simulink model "DT_PID"  (R2025b)
settings: Solver=ode4  StartTime=0.0  StopTime=10.0  FixedStep=0.01  RelTol=1e-3
model workspace (MAT data in the model file):
  K = 126
  tau = 0.1
settings Model: Creator=joshc  LastModifiedBy=joshc

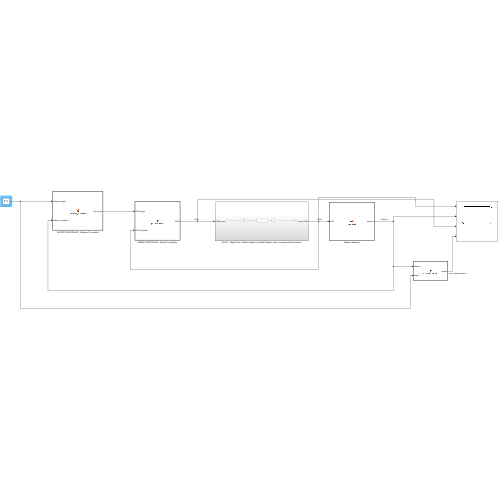
[thumbnail: Simulink's stored preview of the top-level diagram]
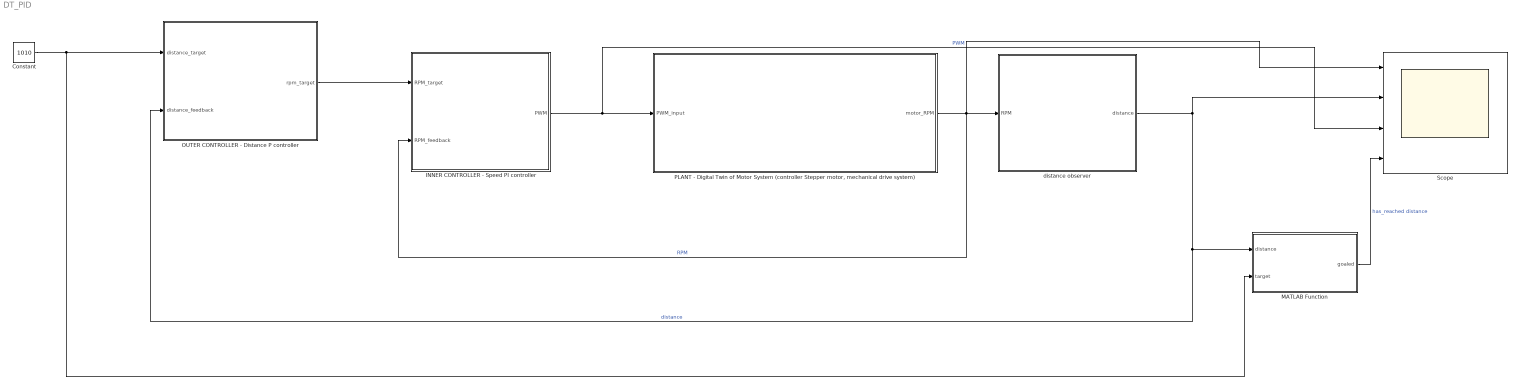
== system DT_PID ==
  Constant : Constant  Value=1010
  INNER CONTROLLER - Speed PI controller : MATLAB Function  TreatAsAtomicUnit=on
  MATLAB Function : MATLAB Function  TreatAsAtomicUnit=on
  OUTER CONTROLLER - Distance P controller : MATLAB Function  TreatAsAtomicUnit=on
  "PLANT - Digital Twin of Motor System (controller Stepper motor, mechanical drive system)" : Subsystem
  Scope : Scope  NumInputPorts=4
      settings: ActiveDisplayYMinimum=-63.762879455181228  ActiveDisplayYMaximum=573.86591509663117
  distance observer : MATLAB Function  TreatAsAtomicUnit=on
  wires:
  INNER CONTROLLER - Speed PI controller/1(PWM) -> Scope/3, "PLANT - Digital Twin of Motor System (controller Stepper motor, mechanical drive system)"/1(PWM_input)  "PWM"
  "PLANT - Digital Twin of Motor System (controller Stepper motor, mechanical drive system)"/1(motor_RPM) -> Scope/1, INNER CONTROLLER - Speed PI controller/2(RPM_feedback), distance observer/1(RPM)  "RPM"
  OUTER CONTROLLER - Distance P controller/1(rpm_target) -> INNER CONTROLLER - Speed PI controller/1(RPM_target)
  distance observer/1(distance) -> Scope/2, MATLAB Function/1(distance), OUTER CONTROLLER - Distance P controller/2(distance_feedback)  "distance"
  MATLAB Function/1(goaled) -> Scope/4  "has_reached distance"
  Constant/1 -> MATLAB Function/2(target), OUTER CONTROLLER - Distance P controller/1(distance_target)

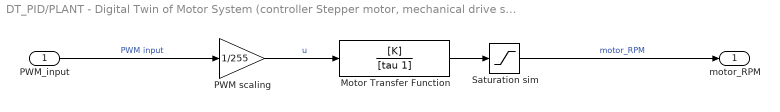
== system DT_PID/PLANT - Digital Twin of Motor System (controller Stepper motor, mechanical drive system) ==
  PWM_input : Inport
  Motor Transfer Function : TransferFcn  Numerator=[K]  Denominator=[tau 1]
  PWM scaling : Gain  Gain=1/255
  Saturation sim : Saturate  UpperLimit=186  LowerLimit=0
  motor_RPM : Outport
  wires:
  PWM_input/1 -> PWM scaling/1  "PWM input"
  PWM scaling/1 -> Motor Transfer Function/1  "u"
  Motor Transfer Function/1 -> Saturation sim/1
  Saturation sim/1 -> motor_RPM/1  "motor_RPM"

== matlab function DT_PID/INNER CONTROLLER - Speed PI controller ==
  settings: updateMethod=DISCRETE
  data: RPM_target input; PWM output; RPM_feedback input
function PWM = pid_controller(RPM_target, RPM_feedback)

Kp = 6;
Ki = 0.002;
Kd = 0.0;
Ts = 0.01;

persistent integral prev_error
if isempty(integral)
    integral = 0;
end

if isempty(prev_error)
    prev_error = 0;
end

error = (RPM_target - RPM_feedback);
integral = integral + error*Ts;
derivative = (error - prev_error);

u = Kp*error + Ki*integral + Kd*derivative;
PWM = min(max(u, 0), 255);

prev_error = error;
end

== matlab function DT_PID/OUTER CONTROLLER - Distance P controller ==
  data: distance_target input; rpm_target output; distance_feedback input
function rpm_target = distance_controller(distance_target, distance_feedback)

Kp_d = 1.2;
Ki_d = 0.0;
Ts = 0.01;

persistent integral_d
if isempty(integral_d)
    integral_d = 0;
end

error_d = (distance_target - distance_feedback);
integral_d = integral_d + error_d*Ts;

rpm_target = Kp_d*error_d + Ki_d*integral_d;

== matlab function DT_PID/MATLAB Function ==
  data: distance input; goaled output; target input
function goaled = distance_check(distance, target)

if distance >= target - (target/200)
    goaled = 100;
else
    goaled = 0;
end

== matlab function DT_PID/distance observer ==
  settings: updateMethod=DISCRETE
  data: RPM input; distance output
function distance = rpm2dist(RPM)

diameter = 49.7;
Ts = 0.01;

circumference = pi*diameter;

persistent x
if isempty(x)
    x = 0;
end

speed = (RPM/60)*circumference;

x = x + speed*Ts;

distance = x;
